simulink model "mbed_disco_f407_display"  (R2015a)
settings: Solver=FixedStepDiscrete  SolverMode=SingleTasking  StartTime=0.0  StopTime=10.0  FixedStep=1e-3  RelTol=1e-3
libraries: simulink x1, LCDScope x1
settings Model: Creator=oh  LastModifiedBy=oh
settings OptimizationCC: OptimizeModelRefInitCode=on  LifeSpan=1
settings HardwareCC: ProdLargestAtomicInteger=Long  ProdLargestAtomicFloat=Double  ProdEndianess=LittleEndian  ProdHWDeviceType=ARM Compatible->ARM Cortex
settings RTWCC: SystemTargetFile=mbed.tlc  TemplateMakefile=mbed.tmf  Description=Mbed Target (Embedded Target)  TargetLang=C++
settings CodeAppCC: IgnoreCustomStorageClasses=off
settings STFCustomTargetCC: CombineOutputUpdateFcns=on  SupportContinuousTime=off  SupportVariableSizeSignals=off  SystemTargetFile=mbed.tlc
settings ERTTargetCC: SupportContinuousTime=off  SupportVariableSizeSignals=off  ERTCustomFileTemplate=mbed_file_process.tlc

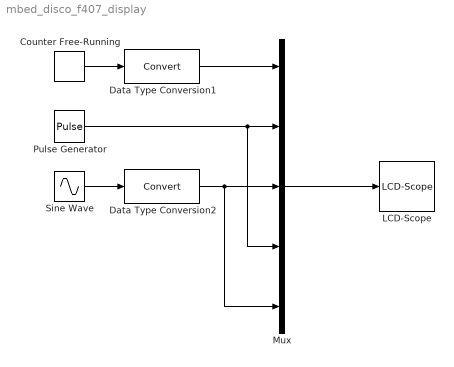
== system mbed_disco_f407_display ==
  Counter Free-Running : simulink/Sources/Counter Free-Running  NumBits=6  tsamp=-1
  Data Type Conversion1 : DataTypeConversion
  Data Type Conversion2 : DataTypeConversion
  LCD-Scope : LCDScope/LCD-Scope  MinValue=0  MaxValue=120  StepSize=1  scaleValue=1e0
      settings: TimeRange=500
  Mux : Mux  Inputs=5
  Pulse Generator : DiscretePulseGenerator  PulseType=Time based  Amplitude=100  Period=10  PulseWidth=5
  Sine Wave : Sin  Amplitude=50  Bias=50
  wires:
  Counter Free-Running/1 -> Data Type Conversion1/1
  Pulse Generator/1 -> Mux/4, Mux/2
  Mux/1 -> LCD-Scope/1
  Data Type Conversion1/1 -> Mux/1
  Sine Wave/1 -> Data Type Conversion2/1
  Data Type Conversion2/1 -> Mux/5, Mux/3
